simulink model "PMSM_generator"  (R2022a)
settings: Solver=ode45  StartTime=0.0  StopTime=stop_time  RelTol=1e-3
values from neighbouring files (symbols this model uses):
  B_eq = param{6}    [measurement_2states.m]    (also in measurement_2states_3mes.m; measurement_3measure.m)
undefined symbols (not defined in the file or in its folder): Gc, gearbox, generator, I_eq, simulation
libraries: slpidlib x1
settings Model: Creator=Niccolò  LastModifiedBy=Niccolò

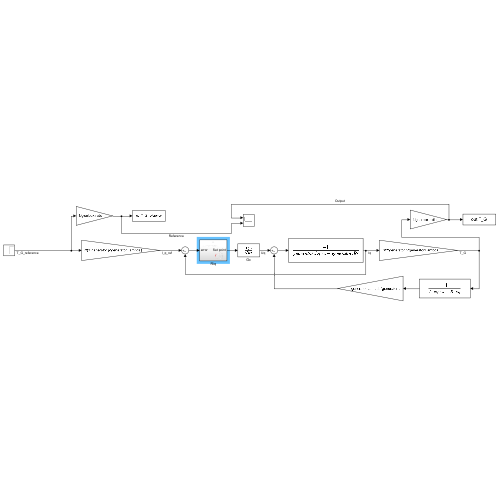
[thumbnail: Simulink's stored preview of the top-level diagram]
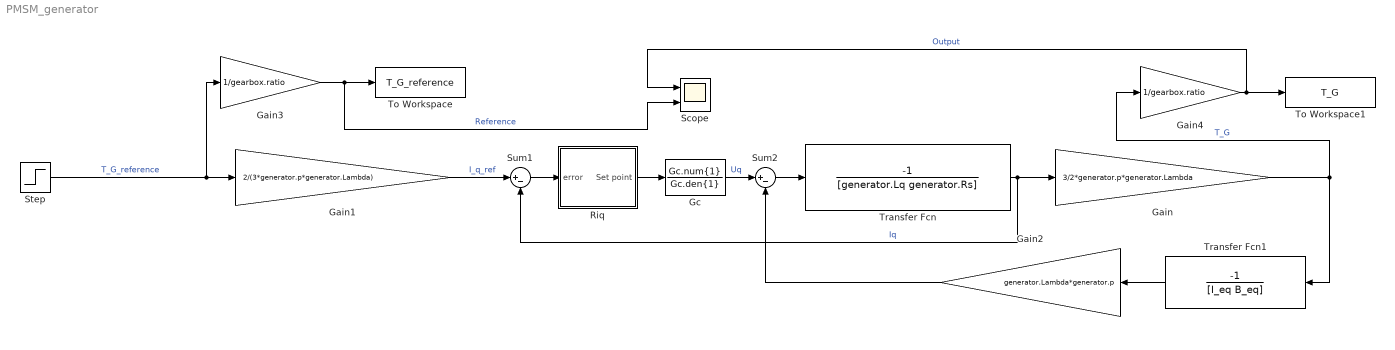
== system PMSM_generator ==
  Gain : Gain  Gain=3/2*generator.p*generator.Lambda  SampleTime=simulation.time_step_L
  Gain1 : Gain  Gain=2/(3*generator.p*generator.Lambda)  SampleTime=simulation.time_step_L
  Gain2 : Gain  Gain=generator.Lambda*generator.p
  Gain3 : Gain  Gain=1/gearbox.ratio
  Gain4 : Gain  Gain=1/gearbox.ratio
  Gc : TransferFcn  Numerator=Gc.num{1}  Denominator=Gc.den{1}
  Riq : Subsystem
  Scope : Scope  NumInputPorts=2
  Step : Step  Time=0.5  SampleTime=0
  Sum1 : Sum  Inputs=|+-  SampleTime=simulation.time_step_L
  Sum2 : Sum  Inputs=|+-
  To Workspace : ToWorkspace  VariableName=T_G_reference  SaveFormat=Timeseries  SampleTime=-1
  To Workspace1 : ToWorkspace  VariableName=T_G  SaveFormat=Timeseries  SampleTime=-1
  Transfer Fcn : TransferFcn  Numerator=[-1]  Denominator=[generator.Lq generator.Rs]
  Transfer Fcn1 : TransferFcn  Numerator=[-1]  Denominator=[I_eq B_eq]
  wires:
  Sum2/1 -> Transfer Fcn/1
  Transfer Fcn/1 -> Sum1/2, Gain/1  "Iq"
  Gain1/1 -> Sum1/1  "I_q_ref"
  Riq/1(Set point) -> Gc/1
  Sum1/1 -> Riq/1(error)
  Gain2/1 -> Sum2/2
  Step/1 -> Gain3/1, Gain1/1  "T_G_reference"
  Gc/1 -> Sum2/1  "Uq"
  Gain/1 -> Transfer Fcn1/1, Gain4/1  "T_G"
  Gain3/1 -> Scope/2, To Workspace/1  "Reference"
  Gain4/1 -> Scope/1, To Workspace1/1  "Output"
  Transfer Fcn1/1 -> Gain2/1

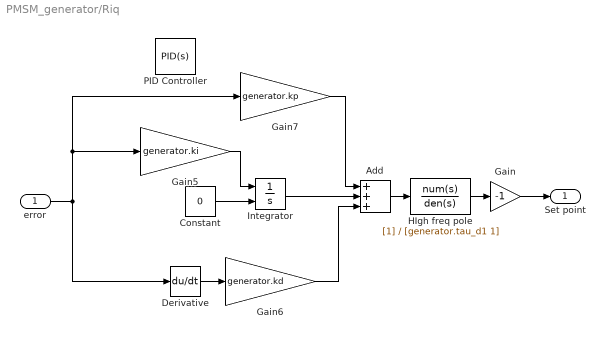
== system PMSM_generator/Riq ==
  error : Inport
  Add : Sum  Inputs=+++
  Constant : Constant  Value=0
  Derivative : Derivative
  Gain : Gain  Gain=-1
  Gain5 : Gain  Gain=generator.ki
  Gain6 : Gain  Gain=generator.kd
  Gain7 : Gain  Gain=generator.kp
  HIgh freq pole : TransferFcn  Denominator=[generator.tau_d1 1]
  Integrator : Integrator  InitialConditionSource=external
  PID Controller : slpidlib/PID Controller  Controller=PID  Form=Parallel  TimeDomain=Continuous-time  UseExternalTs=off  SampleTime=-1  IntegratorMethod=Forward Euler  FilterMethod=Forward Euler  ControllerParametersSource=internal  P=generator.kp  I=generator.ki  UseKiTs=off  D=generator.kd  N=0  UseFilter=on  TunerSelectOption=Transfer Function Based (PID Tuner App)  InitialConditionSource=internal  InitialConditionForIntegrator=0  InitialConditionForFilter=0  DifferentiatorICPrevScaledInput=0  ExternalReset=none  TrackingMode=off  Kt=1  LimitOutput=off  SatLimitsSource=internal  UpperSaturationLimit=inf  LowerSaturationLimit=-inf  LinearizeAsGain=on  AntiWindupMode=none  Kb=1  POutMin=[]  POutMax=[]  IOutMin=[]  IOutMax=[]  DOutMin=[]  DOutMax=[]  NOutMin=[]  NOutMax=[]  SumOutMin=[]  SumOutMax=[]  SaturationOutMin=[]  SaturationOutMax=[]  PParamMin=[]  PParamMax=[]  IParamMin=[]  IParamMax=[]  DParamMin=[]  DParamMax=[]  NParamMin=[]  NParamMax=[]  KbParamMin=[]  KbParamMax=[]  KtParamMin=[]  KtParamMax=[]  KbOutMin=[]  KbOutMax=[]  KtOutMin=[]  KtOutMax=[]  IntegratorOutMin=[]  IntegratorOutMax=[]  FilterOutMin=[]  FilterOutMax=[]  SumI1OutMin=[]  SumI1OutMax=[]  SumI2OutMin=[]  SumI2OutMax=[]  SumI3OutMin=[]  SumI3OutMax=[]  SumI4OutMin=[]  SumI4OutMax=[]  SumDOutMin=[]  SumDOutMax=[]  DifferentiatorOutMin=[]  DifferentiatorOutMax=[]  FilterDiffOutCoefMin=[]  FilterDiffOutCoefMax=[]  ReciprocalOutMin=[]  ReciprocalOutMax=[]  SumDenOutMin=[]  SumDenOutMax=[]  SumNumOutMin=[]  SumNumOutMax=[]  DivideOutMin=[]  DivideOutMax=[]  UdiffTsProdOutMin=[]  UdiffTsProdOutMax=[]  NTsProdOutMin=[]  NTsProdOutMax=[]  UintegralTsProdOutMin=[]  UintegralTsProdOutMax=[]  UngainTsProdOutMin=[]  UngainTsProdOutMax=[]  IntegratorContinuousStateAttributes=''  IntegratorStateMustResolveToSignalObject=off  IntegratorRTWStateStorageClass=Auto  FilterContinuousStateAttributes=''  FilterStateMustResolveToSignalObject=off  FilterRTWStateStorageClass=Auto  ParallelPVariant=InternalParameters  IdealPVariant=Disabled  IVariant=InternalParameters  DVariant=InternalParameters  IntegratorVariant=Continuous  SatVariant=Disabled  AWVariant=Passthrough  PCopyVariant=Disabled  TRVariant=Disabled  FdbkBlocksVariant=Forward  IdealPFdbkVariant=Disabled  SatFdbkVariant=Disabled  DerivativeFilterVariant=ContFilter  NVariant=InternalParameters  NCopyVariant=Disabled  FilterICVariant=InternalICsFilter  IntegratorICVariant=InternalICs  ExternalResetVariant=Disabled  TRSumVariant=Passthrough  SumFdbkVariant=Disabled  SumVariant=Sum_PID  TsampFilterVariant=InternalTs  TsampNgainVariant=Passthrough  TsampIntegralVariant=Passthrough  ExternalSaturationOutDataTypeStr=Inherit: Same as second input  aMode=0
  Set point : Outport
  wires:
  Gain/1 -> Set point/1
  HIgh freq pole/1 -> Gain/1
  Gain5/1 -> Integrator/1
  Constant/1 -> Integrator/2
  Derivative/1 -> Gain6/1
  Gain6/1 -> Add/3
  Gain7/1 -> Add/1
  Integrator/1 -> Add/2
  error/1 -> Derivative/1, Gain5/1, Gain7/1
  Add/1 -> HIgh freq pole/1
